simulink model "FCW_Simulink"  (R2022b)
settings: Solver=VariableStepAuto  StartTime=0.0  StopTime=53  RelTol=1e-3
settings Model: Creator=adamg  LastModifiedBy=adamg

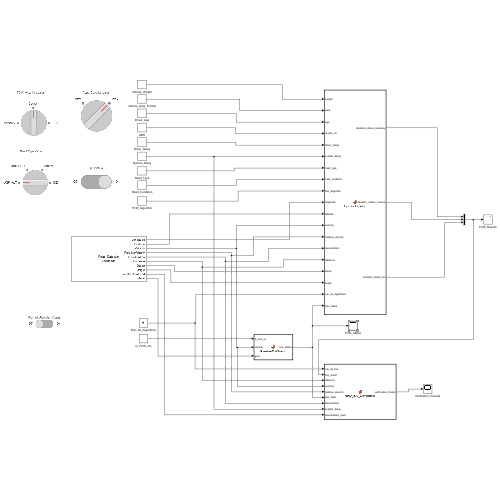
[thumbnail: Simulink's stored preview of the top-level diagram]
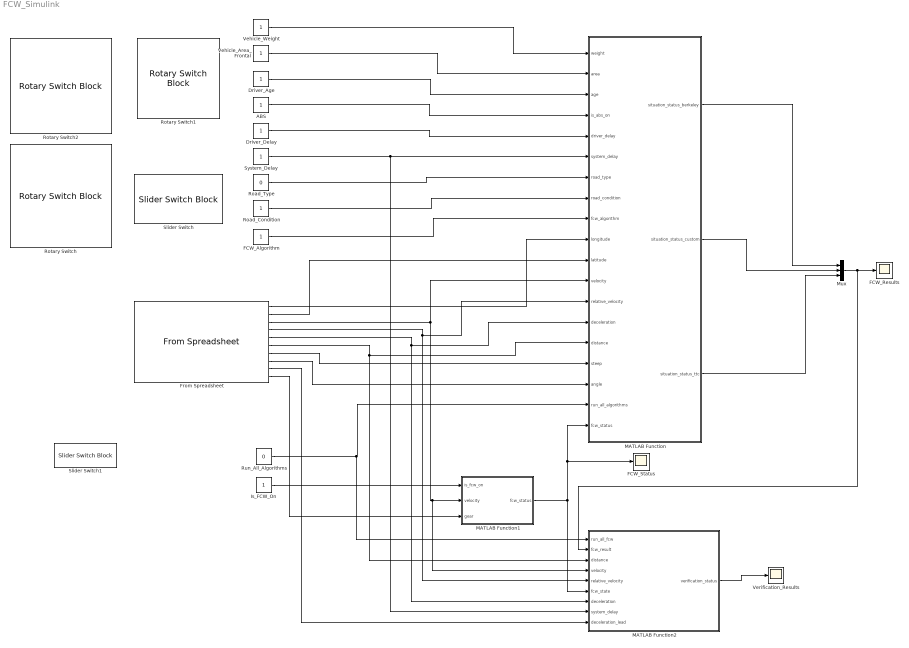
== system FCW_Simulink ==
  ABS : Constant
  Driver_Age : Constant
  Driver_Delay : Constant
  FCW_Algorithm : Constant
  FCW_Results : Scope
  FCW_Status : Scope
  From Spreadsheet : FromSpreadsheet  FileName=Road_Data.xlsx  SheetName=Scenario5  Range=A1:K54  ExtrapolationBeforeFirstDataPoint=Hold first value  ExtrapolationAfterLastDataPoint=Hold last value
  Is_FCW_On : Constant
  MATLAB Function : MATLAB Function  TreatAsAtomicUnit=on
  MATLAB Function1 : MATLAB Function  TreatAsAtomicUnit=on
  MATLAB Function2 : MATLAB Function  TreatAsAtomicUnit=on
  Mux : Mux  Inputs=3
  Road_Condition : Constant
  Road_Type : Constant  Value=0
  Rotary Switch : RotarySwitchBlock  UseEnumeratedDataType=on  EnumeratedDataType=Road_Type
      settings: Values={{'ASPHALT', 'CONCRETE', 'SNOW', 'ICE'}, [0 1 2 3]}
  Rotary Switch1 : RotarySwitchBlock  UseEnumeratedDataType=on  EnumeratedDataType=Road_Condition
      settings: Values={{'WET', 'DRY'}, [0 1]}
  Rotary Switch2 : RotarySwitchBlock
      settings: Values={{'Berkeley', 'Custom', 'TTC'}, [0 1 2]}
  Run_All_Algorithms : Constant  Value=0
  Slider Switch : SliderSwitchBlock
      settings: Values={{'Off', 'On'}, [0 1]}
  Slider Switch1 : SliderSwitchBlock
      settings: Values={{'Off', 'On'}, [0 1]}
  System_Delay : Constant
  Vehicle_Area_Frontal : Constant
  Vehicle_Weight : Constant
  Verification_Results : Scope
  wires:
  Vehicle_Weight/1 -> MATLAB Function/1(weight)
  Vehicle_Area_Frontal/1 -> MATLAB Function/2(area)
  Driver_Age/1 -> MATLAB Function/3(age)
  ABS/1 -> MATLAB Function/4(is_abs_on)
  Driver_Delay/1 -> MATLAB Function/5(driver_delay)
  System_Delay/1 -> MATLAB Function/6(system_delay), MATLAB Function2/8(system_delay)
  Road_Type/1 -> MATLAB Function/7(road_type)
  Road_Condition/1 -> MATLAB Function/8(road_condition)
  FCW_Algorithm/1 -> MATLAB Function/9(fcw_algorithm)
  From Spreadsheet/1 -> MATLAB Function/10(longitude)
  From Spreadsheet/2 -> MATLAB Function/11(latitude)
  From Spreadsheet/3 -> MATLAB Function2/4(velocity), MATLAB Function1/2(velocity), MATLAB Function/12(velocity)
  From Spreadsheet/5 -> MATLAB Function2/7(deceleration), MATLAB Function/14(deceleration)
  From Spreadsheet/6 -> MATLAB Function2/3(distance), MATLAB Function/15(distance)
  From Spreadsheet/7 -> MATLAB Function/16(steep)
  From Spreadsheet/8 -> MATLAB Function/17(angle)
  MATLAB Function/1(situation_status_berkeley) -> Mux/1
  From Spreadsheet/4 -> MATLAB Function2/5(relative_velocity), MATLAB Function/13(relative_velocity)
  Run_All_Algorithms/1 -> MATLAB Function2/1(run_all_fcw), MATLAB Function/18(run_all_algorithms)
  MATLAB Function/2(situation_status_custom) -> Mux/2
  MATLAB Function/3(situation_status_ttc) -> Mux/3
  Mux/1 -> MATLAB Function2/2(fcw_result), FCW_Results/1
  Is_FCW_On/1 -> MATLAB Function1/1(is_fcw_on)
  MATLAB Function1/1(fcw_status) -> MATLAB Function2/6(fcw_state), FCW_Status/1, MATLAB Function/19(fcw_status)
  MATLAB Function2/1(verification_status) -> Verification_Results/1
  From Spreadsheet/10 -> MATLAB Function1/3(gear)
  From Spreadsheet/9 -> MATLAB Function2/9(deceleration_lead)

== matlab function FCW_Simulink/MATLAB Function1 ==
  data: is_fcw_on input; fcw_status output; velocity input; gear input
function fcw_status = ResolveFCWStatus(is_fcw_on, velocity, gear)

fcw_status = -1;

coder.extrinsic("FCW_Assistant_Status");

fcw_status = FCW_Assistant_Status(is_fcw_on, velocity, gear);

== matlab function FCW_Simulink/MATLAB Function ==
  data: weight input; situation_status_berkeley output; area input; age input; is_abs_on input; driver_delay input; system_delay input; road_type input; road_condition input; fcw_algorithm input; longitude input; latitude input; velocity input; relative_velocity input; deceleration input; distance input; steep input; angle input; run_all_algorithms input; situation_status_custom output; situation_status_ttc output; fcw_status input
function [situation_status_berkeley, situation_status_custom, situation_status_ttc] = ResolveSituation(weight, area, age, is_abs_on, driver_delay, system_delay, road_type, road_condition, fcw_algorithm, ...
    longitude, latitude, velocity, relative_velocity, deceleration, distance, steep, angle, run_all_algorithms, fcw_status)

situation_status_berkeley = 2;
situation_status_custom = 2;
situation_status_ttc = 2;

coder.extrinsic("FCW_Matlab_Main");

if fcw_status == 1 % if FCW Assistant is ACTIVE

    situation_statuses = [FCW_Matlab_Main(weight, area, age, is_abs_on, driver_delay, system_delay, road_type, road_condition, fcw_algorithm, ...
        longitude, latitude, velocity, relative_velocity, deceleration, distance, steep, angle, run_all_algorithms)];
    
    if run_all_algorithms == 1
        situation_status_berkeley = double(situation_statuses(1));
        situation_status_custom = double(situation_statuses(2));
        situation_status_ttc = double(situation_statuses(3));
    else
        if fcw_algorithm == 0
            situation_status_berkeley = double(situation_statuses(1));
        elseif fcw_algorithm == 1
             situation_status_custom = double(situation_statuses(1));
        elseif fcw_algorithm == 2
             situation_status_ttc = double(situation_statuses(1));
        else
            error("Unsupported FCW algorithm!");
        end
    end
end


%situation_status = double(FCW_Matlab_Main(weight, area, age, is_abs_on, driver_delay, system_delay, road_type, road_condition, fcw_algorithm, ...
%    longitude, latitude, velocity, relative_velocity, deceleration, distance, steep, angle, run_all_algorithms));

== matlab function FCW_Simulink/MATLAB Function2 ==
  data: run_all_fcw input; fcw_result input; verification_status output; distance input; velocity input; relative_velocity input; fcw_state input; deceleration input; system_delay input; deceleration_lead input
function verification_status = Verify_ISO_Compliance(run_all_fcw, fcw_result, distance, velocity, relative_velocity, fcw_state, deceleration, system_delay, deceleration_lead)
verification_status = -1;

%disp(fcw_result);

coder.extrinsic("FCW_ISO_Verification");

min_distance = 10;  % in m

if run_all_fcw == 0 
    
    if fcw_result(1) ~= 2
        selected_fcw_result = fcw_result(1);
    elseif fcw_result(2) ~= 2
        selected_fcw_result = fcw_result(2);
    else
        selected_fcw_result = fcw_result(3);
    end
    
    verification_status = FCW_ISO_Verification(selected_fcw_result, distance, velocity, relative_velocity, fcw_state, deceleration, min_distance, system_delay, deceleration_lead);
end
